simulink model "ECE453_Hw9"  (R2025a)
settings: Solver=VariableStepAuto  StartTime=0.0  StopTime=0.1  RelTol=1e-3
model workspace (MAT data in the model file):
  Vdc = 200
libraries: spsTriangleGeneratorLib x1
settings Model: Creator=cruisemac  LastModifiedBy=cruisemac

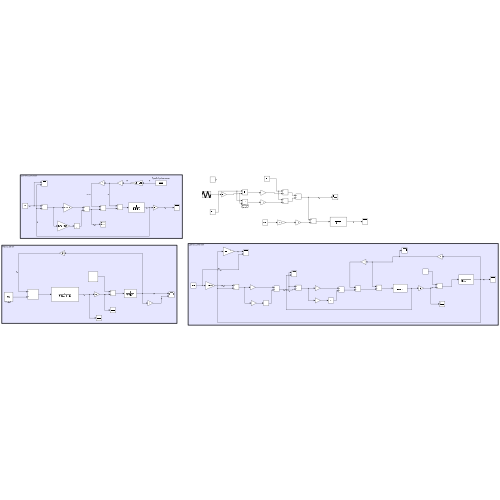
[thumbnail: Simulink's stored preview of the top-level diagram]
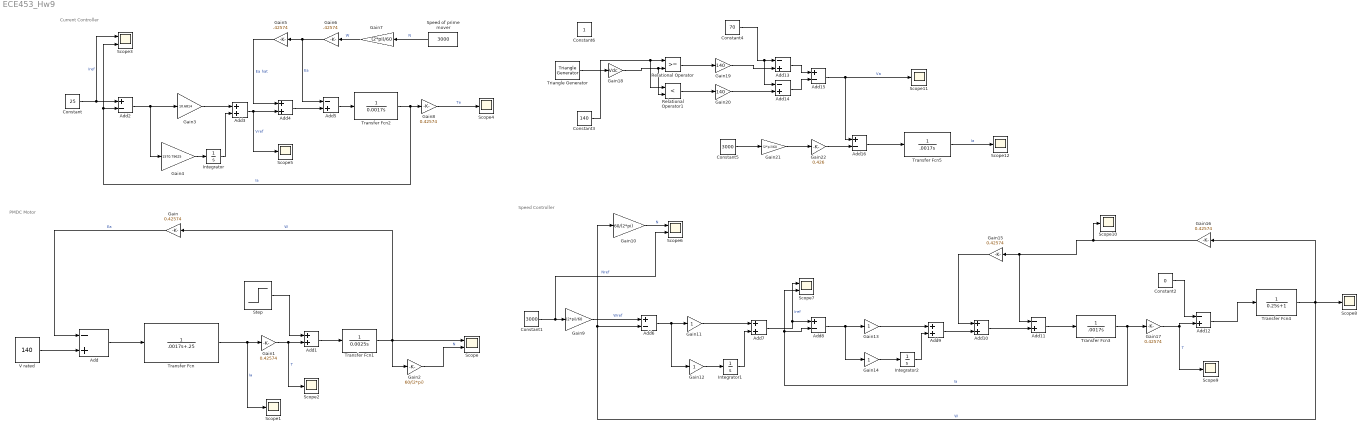
== system ECE453_Hw9 ==
  note: Speed Controller
  note: Current Controller
  note: PMDC Motor
  Add{,5,11..14} (6 alike) : Sum  Inputs=-+
  Add{1,3..4,7,9..10} (6 alike) : Sum
  Add{2,6,8,15..16} (5 alike) : Sum  Inputs=+-
  Constant : Constant  Value=25
  Constant1 : Constant  Value=3000
  Constant2 : Constant  Value=0
  Constant3 : Constant  Value=140
  Constant4 : Constant  Value=70
  Constant5 : Constant  Value=3000
  Constant6 : Constant
  Gain{,1,8,15..17} (6 alike) : Gain  Gain=0.42574
  Gain10 : Gain  Gain=60/(2*pi)
  Gain{11..14} (4 alike) : Gain
  Gain18 : Gain  Gain=Vdc
  Gain19 : Gain  Gain=140
  Gain2 : Gain  Gain=60/(2*pi)
  Gain20 : Gain  Gain=140
  Gain21 : Gain  Gain=(2*pi)/60
  Gain22 : Gain  Gain=0.426
  Gain3 : Gain  Gain=10.6814
  Gain4 : Gain  Gain=1570.79625
  Gain5 : Gain  Gain=.42574
  Gain6 : Gain  Gain=.42574
  Gain7 : Gain  Gain=(2*pi)/60
  Gain9 : Gain  Gain=(2*pi)/60
  Integrator : Integrator
  Integrator1 : Integrator
  Integrator2 : Integrator
  Relational Operator : RelationalOperator  OutDataTypeStr=boolean  RndMeth=Simplest  InputSameDT=off
  Relational Operator1 : RelationalOperator  Operator=<  OutDataTypeStr=boolean  RndMeth=Simplest  InputSameDT=off
  Scope{,3,6..7} (4 alike) : Scope  NumInputPorts=2
      Scope settings: ActiveDisplayYMinimum=-231.47716176190852  ActiveDisplayYMaximum=5264.99250503524
      Scope3 settings: ActiveDisplayYMinimum=-4.1909869617950264  ActiveDisplayYMaximum=28.621513038204974  DataLoggingVariableName=ScopeData3
      Scope6 settings: DataLoggingVariableName=ScopeData6
      Scope7 settings: ActiveDisplayYMinimum=-39.295130247450295  ActiveDisplayYMaximum=353.65617222705271  DataLoggingVariableName=ScopeData7
  Scope{1..2,4..5,8..12} (9 alike) : Scope
      Scope1 settings: ActiveDisplayYMinimum=-1  ActiveDisplayYMaximum=1
      Scope10 settings: ActiveDisplayYMinimum=-16.536592700020449  ActiveDisplayYMaximum=67.352675866905784  DataLoggingVariableName=ScopeData10
      Scope11 settings: ActiveDisplayYMinimum=-9.67694208388994  ActiveDisplayYMaximum=180.29331355544977  DataLoggingVariableName=ScopeData11
      Scope12 settings: ActiveDisplayYMinimum=-1  ActiveDisplayYMaximum=1  DataLoggingVariableName=ScopeData12
      Scope2 settings: DataLoggingVariableName=ScopeData2
      Scope4 settings: ActiveDisplayYMinimum=-1  ActiveDisplayYMaximum=1  DataLoggingVariableName=ScopeData4
      Scope5 settings: ActiveDisplayYMinimum=266.83529798906108  ActiveDisplayYMaximum=267.24814090432255  DataLoggingVariableName=ScopeData5
      Scope8 settings: ActiveDisplayYMinimum=-16.536592700020449  ActiveDisplayYMaximum=67.352675866905784  DataLoggingVariableName=ScopeData8
      Scope9 settings: ActiveDisplayYMinimum=-16.606463906037934  ActiveDisplayYMaximum=149.45817515434143  DataLoggingVariableName=ScopeData9
  Speed of prime mover : Constant  Value=3000
  Step : Step  After=10.6424  SampleTime=0
  Transfer Fcn : TransferFcn  Denominator=[.0017 .25]
  Transfer Fcn1 : TransferFcn  Denominator=[0.0025 0]
  Transfer Fcn2 : TransferFcn  Denominator=[0.0017 0]
  Transfer Fcn3 : TransferFcn  Denominator=[.0017 0]
  Transfer Fcn4 : TransferFcn  Denominator=[0.25 1]
  Transfer Fcn5 : TransferFcn  Denominator=[.0017 0]
  Triangle Generator : spsTriangleGeneratorLib/Triangle Generator  Freq=1e3  Phase=90  Ts=0
  V rated : Constant  Value=140
  wires:
  Gain/1 -> Add/1  "Ea"
  Gain1/1 -> Add1/2, Scope2/1  "T"
  Add/1 -> Transfer Fcn/1
  Step/1 -> Add1/1
  Add1/1 -> Transfer Fcn1/1
  Transfer Fcn1/1 -> Gain2/1, Gain/1, Scope/1  "W"
  Gain2/1 -> Scope/2  "N"
  Transfer Fcn/1 -> Gain1/1, Scope1/1  "Ia"
  V rated/1 -> Add/2
  Constant/1 -> Add2/1, Scope3/1  "Iref"
  Add4/1 -> Add5/2
  Transfer Fcn2/1 -> Gain8/1, Add2/2, Scope3/2  "Ia"
  Gain5/1 -> Add4/1  "Ea hat"
  Gain3/1 -> Add3/1
  Add3/1 -> Add4/2, Scope5/1  "Vref"
  Gain7/1 -> Gain6/1  "W"
  Integrator/1 -> Add3/2
  Gain6/1 -> Add5/1, Gain5/1  "Ea"
  Speed of prime mover/1 -> Gain7/1  "N"
  Gain8/1 -> Scope4/1  "Te"
  Add2/1 -> Gain4/1, Gain3/1
  Gain4/1 -> Integrator/1
  Add5/1 -> Transfer Fcn2/1
  Gain16/1 -> Scope10/1, Gain15/1, Add11/1
  Gain15/1 -> Add10/1
  Gain9/1 -> Add6/1  "Wref"
  Add7/1 -> Scope7/1, Add8/1  "Iref"
  Integrator1/1 -> Add7/2
  Add12/1 -> Transfer Fcn4/1
  Add8/1 -> Gain13/1, Gain14/1
  Transfer Fcn4/1 -> Add6/2, Gain10/1, Gain16/1, Scope8/1  "W"
  Gain14/1 -> Integrator2/1
  Gain10/1 -> Scope6/1  "N"
  Gain13/1 -> Add9/1
  Constant1/1 -> Gain9/1, Scope6/2  "Nref"
  Add9/1 -> Add10/2
  Add10/1 -> Add11/2
  Gain17/1 -> Add12/2, Scope9/1  "T"
  Gain11/1 -> Add7/1
  Constant2/1 -> Add12/1
  Add11/1 -> Transfer Fcn3/1
  Add6/1 -> Gain11/1, Gain12/1
  Gain12/1 -> Integrator1/1
  Integrator2/1 -> Add9/2
  Transfer Fcn3/1 -> Scope7/2, Add8/2, Gain17/1  "Ia"
  Add13/1 -> Add15/1
  Add15/1 -> Add16/1, Scope11/1  "Va"
  Relational Operator1/1 -> Gain20/1
  Transfer Fcn5/1 -> Scope12/1  "Ia"
  Gain20/1 -> Add14/2
  Add16/1 -> Transfer Fcn5/1
  Gain21/1 -> Gain22/1
  Add14/1 -> Add15/2
  Constant5/1 -> Gain21/1
  Relational Operator/1 -> Gain19/1
  Gain19/1 -> Add13/2
  Constant4/1 -> Add13/1, Add14/1
  Gain18/1 -> Relational Operator1/2, Relational Operator/2
  Gain22/1 -> Add16/2
  Constant3/1 -> Relational Operator/1, Relational Operator1/1
  Triangle Generator/1 -> Gain18/1
